simulink model "RCcircuit"  (R2018a)
settings: Solver=ode45  StartTime=0.0  StopTime=2.0  MaxStep=0.01  RelTol=1e-3
undefined symbols (not defined in the file): C, R
settings Model: Creator=Guestmit  LastModifiedBy=Guestmit

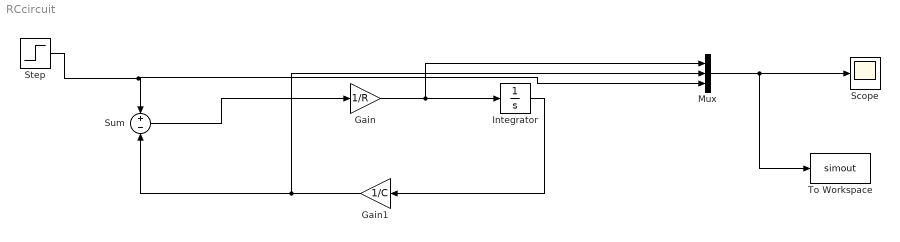
== system RCcircuit ==
  Gain : Gain  Gain=1/R
  Gain1 : Gain  Gain=1/C
  Integrator : Integrator
  Mux : Mux  Inputs=3
  Scope : Scope
  Step : Step  SampleTime=0
  Sum : Sum  Inputs=+-
  To Workspace : ToWorkspace  VariableName=simout  SaveFormat=Timeseries  SampleTime=-1
  wires:
  Step/1 -> Mux/3, Sum/1
  Sum/1 -> Gain/1
  Gain/1 -> Mux/1, Integrator/1
  Integrator/1 -> Gain1/1
  Gain1/1 -> Mux/2, Sum/2
  Mux/1 -> To Workspace/1, Scope/1
